simulink model "planar_vtol_sim"  (R2018a)
settings: Solver=ode45  StartTime=0.0  StopTime=10000  MaxStep=0.1  RelTol=1e-3
undefined symbols (not defined in the file or in its folder): planar_vtol_animation
libraries: simulink x4
settings Model: Creator=canla  LastModifiedBy=canla
settings OptimizationCC: LifeSpan=inf

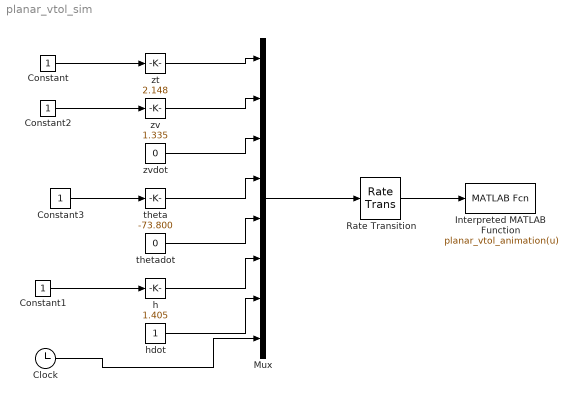
== system planar_vtol_sim ==
  Clock : Clock
  Constant{,1..3} (4 alike) : Constant
  Interpreted MATLAB Function : MATLABFcn  MATLABFcn=planar_vtol_animation(u)  OutputDimensions=-0
  Mux : Mux  Inputs=8
  Rate Transition : RateTransition  OutPortSampleTime=P.t_plot
  h : simulink/Math Operations/Slider Gain  gain=1.405  low=0.25  high=3.75
  hdot : Constant
  theta : simulink/Math Operations/Slider Gain  gain=-73.800  low=-90  high=90
  thetadot : Constant  Value=0
  zt : simulink/Math Operations/Slider Gain  gain=2.148  low=0.15  high=3.85
  zv : simulink/Math Operations/Slider Gain  gain=1.335  low=0.25  high=3.75
  zvdot : Constant  Value=0
  wires:
  Mux/1 -> Rate Transition/1
  Constant/1 -> zt/1
  zt/1 -> Mux/1
  zv/1 -> Mux/2
  Constant2/1 -> zv/1
  zvdot/1 -> Mux/3
  theta/1 -> Mux/4
  thetadot/1 -> Mux/5
  h/1 -> Mux/6
  Constant1/1 -> h/1
  hdot/1 -> Mux/7
  Rate Transition/1 -> Interpreted MATLAB Function/1
  Clock/1 -> Mux/8
  Constant3/1 -> theta/1
